simulink model "comparetoconstant_complex_test"  (Simulink 8.4)
settings: Solver=ode45  StartTime=0.0  StopTime=10.0  RelTol=1e-3
libraries: simulink x5
settings Model: Creator=arnaud  LastModifiedBy=arnaud
settings DataIOCC: SaveFormat=Structure  SignalLoggingSaveFormat=Dataset
settings OptimizationCC: ExpressionDepthLimit=128
settings DebuggingCC: UnderspecifiedInitializationDetection=Simplified  MergeDetectMultiDrivingBlocksExec=error  FcnCallInpInsideContextMsg=EnableAllAsError  StateNameClashWarn=none
settings GRTTargetCC: CombineOutputUpdateFcns=on  GRTInterface=off

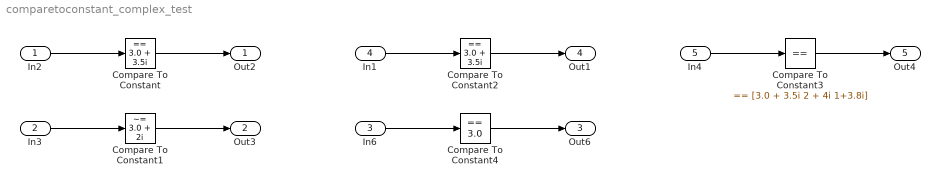
== system comparetoconstant_complex_test ==
  In2 : Inport  OutDataTypeStr=double
      settings: SignalType=complex
  In3 : Inport  Port=2  OutDataTypeStr=int8
      settings: SignalType=complex
  In6 : Inport  Port=3  OutDataTypeStr=int8  PortDimensions=3
      settings: SignalType=complex
  In1 : Inport  Port=4  OutDataTypeStr=double  PortDimensions=3
      settings: SignalType=complex
  In4 : Inport  Port=5  OutDataTypeStr=double  PortDimensions=3
      settings: SignalType=complex
  Compare To Constant : simulink/Logic and Bit Operations/Compare To Constant  relop===  const=3.0 + 3.5i  OutDataTypeStr=boolean
  Compare To Constant1 : simulink/Logic and Bit Operations/Compare To Constant  relop=~=  const=3.0 + 2i  OutDataTypeStr=boolean
  Compare To Constant2 : simulink/Logic and Bit Operations/Compare To Constant  relop===  const=3.0 + 3.5i  OutDataTypeStr=boolean
  Compare To Constant3 : simulink/Logic and Bit Operations/Compare To Constant  relop===  const=[3.0 + 3.5i 2 + 4i 1+3.8i]  OutDataTypeStr=boolean
  Compare To Constant4 : simulink/Logic and Bit Operations/Compare To Constant  relop===  const=3.0  OutDataTypeStr=boolean
  Out2 : Outport
  Out3 : Outport  Port=2
  Out6 : Outport  Port=3
  Out1 : Outport  Port=4
  Out4 : Outport  Port=5
  wires:
  Compare To Constant/1 -> Out2/1
  In2/1 -> Compare To Constant/1
  Compare To Constant1/1 -> Out3/1
  In3/1 -> Compare To Constant1/1
  Compare To Constant4/1 -> Out6/1
  In6/1 -> Compare To Constant4/1
  Compare To Constant2/1 -> Out1/1
  In1/1 -> Compare To Constant2/1
  Compare To Constant3/1 -> Out4/1
  In4/1 -> Compare To Constant3/1
